simulink model "safir_a"  (R2012b)
(part 2 of 48)

      | port_label('input', 1, 'd');
      | port_label('output', 1, 'q');
      | disp(['Z^-', num2str(latency)]);
  pipeline77 : Subsystem  AncestorBlock=casper_library_delays/pipeline  mask(pipeline){latency=2}
      mask help:
      | An explicitly laid-out delay line to avoid mapping to SRL16s
      | for use in pipelining to help achieve timing closure.
      mask init:
      | pipeline_init(gcb,'latency',latency);
      settings: AttributesFormatString=Latency = %<latency>
      mask Display:
      | port_label('input', 1, 'd');
      | port_label('output', 1, 'q');
      | disp(['Z^-', num2str(latency)]);
  pipeline8 : Subsystem  AncestorBlock=casper_library_delays/pipeline  mask(pipeline){latency=2}
      mask help:
      | An explicitly laid-out delay line to avoid mapping to SRL16s
      | for use in pipelining to help achieve timing closure.
      mask init:
      | pipeline_init(gcb,'latency',latency);
      settings: AttributesFormatString=Latency = %<latency>
      mask Display:
      | port_label('input', 1, 'd');
      | port_label('output', 1, 'q');
      | disp(['Z^-', num2str(latency)]);
  pipeline9 : Subsystem  AncestorBlock=casper_library_delays/pipeline  mask(pipeline){latency=2}
      mask help:
      | An explicitly laid-out delay line to avoid mapping to SRL16s
      | for use in pipelining to help achieve timing closure.
      mask init:
      | pipeline_init(gcb,'latency',latency);
      settings: AttributesFormatString=Latency = %<latency>
      mask Display:
      | port_label('input', 1, 'd');
      | port_label('output', 1, 'q');
      | disp(['Z^-', num2str(latency)]);
  receptor_id : Subsystem  Tag=xps:sw_reg  AncestorBlock=xps_library/software register  mask(swreg){mode=fields of arbitrary size, io_dir=From Processor, io_delay=1, sample_period=1, names=[receptor_id pol0_id pol1_id], bitwidths=[14 2 2], arith_types=[0 0 0], bin_pts=[0 0 0], show_format=on}
      mask prompts: io_dir "I/O direction"; io_delay "I/O delay"; sample_period "Sample period"; names "Names [msb ... lsb]:"; bitwidths "Bitwidths [msb ... lsb]:"; arith_types "Types (ufix=0, fix=1, bool=2) [msb ... lsb]:"; bin_pts "Binary pts [msb ... lsb]:"; show_format "Print format string?"
      mask init:
      | swreg_init(gcb)
      settings: AttributesFormatString=3 inputs:uf14.0,uf2.0,uf2.0,
      mask TypeOptions mode: one value | fields of equal size | fields of arbitrary size
      mask Callback mode: swreg_cb(gcb);
      mask TypeOptions io_dir: To Processor | From Processor
      mask Callback io_dir:
      | mask_enables = get_param(gcb, 'MaskEnables');
      | mask_names = get_param(gcb, 'MaskNames');
      | if strcmp(get_param(gcb, 'io_dir'), 'To Processor'),
      |     mask_enables{ismember(mask_names, 'sample_period')} = 'off';
      | else
      |     mask_enables{ismember(mask_names, 'sample_period')} = 'on';
      | end
      | set_param(gcb, 'MaskEnables', mask_enables);
      mask Callback bitwidths:
      | blk = gcb;
      | mode = get_param(blk, 'mode');
      | current_widths = eval(get_param(blk, 'bitwidths'));
      | if (strcmp(mode, 'one value') || strcmp(mode, 'fields of equal size')) && (length(current_widths) > 1),
      |     error('Only one width may be specified for this mode.');
      | elseif strcmp(mode, 'fields of arbitrary size')
      |     current_names = textscan(strtrim(strrep(strrep(get_param(blk, 'names'), ']', ''), '[', '')), '%s');
      |     current_names = current_names{1};
      |     numios = length(current_names);
      |     if length(current_widths) ~= numios,
      |         error('%d field names specified, but %d widths?', numios, length(current_widths));
      |     end
      | end
      | total_width = 0;
      | for ctr = 1 : length(current_widths),
      |     total_width = total_width + current_widths(ctr);
      | end
      | if total_width > 32,
      |     error('Total width must be 32 or less, set to %d.', total_width);
      | end
      mask Callback arith_types:
      | blk = gcb;
      | mode = get_param(blk, 'mode');
      | current_types = eval(get_param(blk, 'arith_types'));
      | numios = length(current_types);
      | if (strcmp(mode, 'one value') || strcmp(mode, 'fields of equal size')) && (length(current_types) > 1),
      |     error('Only one type may be specified for this mode.');
      | elseif strcmp(mode, 'fields of arbitrary size')
      |     current_names = textscan(strtrim(strrep(strrep(get_param(blk, 'names'), ']', ''), '[', '')), '%s');
      |     current_names = current_names{1};
      |     numios = length(current_names);
      |     if length(current_types) ~= numios,
      |         error('%d field names specified, but %d types?', numios, length(current_types));
      |     end
      | end
      | problem = 0;
      | for ctr = 1 : numios,
      |     t = current_types(ctr);
      |     if (t < 0) || (t > 2),
      |         problem = t;
      |         ctr = numios + 1;
      |     end
      | end
      | if problem ~= 0,
      |     error('Type cannot be %i, must be 0, 1 or 2.', problem);
      | end
      mask Callback bin_pts:
      | blk = gcb;
      | mode = get_param(blk, 'mode');
      | current_bins = eval(get_param(blk, 'bin_pts'));
      | if (strcmp(mode, 'one value') || strcmp(mode, 'fields of equal size')) && (length(current_bins) > 1),
      |     error('Only one binary pt may be specified for this mode.');
      | elseif strcmp(mode, 'fields of arbitrary size')
      |     current_names = textscan(strtrim(strrep(strrep(get_param(blk, 'names'), ']', ''), '[', '')), '%s');
      |     current_names = current_names{1};
      |     numios = length(current_names);
      |     if length(current_bins) ~= numios,
      |         error('%d field names specified, but %d binary pts?', numios, length(current_bins));
      |     end
      | end
  recverr_ctr : Subsystem  Tag=xps:sw_reg  AncestorBlock=xps_library/software register  mask(swreg){mode=fields of equal size, io_dir=To Processor, io_delay=0, sample_period=1, names=[p0 p1], bitwidths=16, arith_types=0, bin_pts=0, sim_port=off, show_format=on}
      mask prompts: io_dir "I/O direction"; io_delay "I/O delay"; sample_period "Sample period"; names "Names [msb ... lsb]:"; bitwidths "Bitwidth:"; arith_types "Type (ufix=0, fix=1, bool=2):"; bin_pts "Binary pt:"; sim_port "Provide sim input/output?"; show_format "Print format string?"
      mask init:
      | swreg_init(gcb)
      settings: AttributesFormatString=2 outputs:uf16.0,uf16.0,
      mask TypeOptions mode: one value | fields of equal size | fields of arbitrary size
      mask Callback mode: swreg_cb(gcb);
      mask TypeOptions io_dir: To Processor | From Processor
      mask Callback io_dir:
      | mask_enables = get_param(gcb, 'MaskEnables');
      | mask_names = get_param(gcb, 'MaskNames');
      | if strcmp(get_param(gcb, 'io_dir'), 'To Processor'),
      |     mask_enables{ismember(mask_names, 'sample_period')} = 'off';
      | else
      |     mask_enables{ismember(mask_names, 'sample_period')} = 'on';
      | end
      | set_param(gcb, 'MaskEnables', mask_enables);
      mask Callback bitwidths:
      | blk = gcb;
      | mode = get_param(blk, 'mode');
      | current_widths = eval(get_param(blk, 'bitwidths'));
      | if (strcmp(mode, 'one value') || strcmp(mode, 'fields of equal size')) && (length(current_widths) > 1),
      |     error('Only one width may be specified for this mode.');
      | elseif strcmp(mode, 'fields of arbitrary size')
      |     current_names = textscan(strtrim(strrep(strrep(get_param(blk, 'names'), ']', ''), '[', '')), '%s');
      |     current_names = current_names{1};
      |     numios = length(current_names);
      |     if length(current_widths) ~= numios,
      |         error('%d field names specified, but %d widths?', numios, length(current_widths));
      |     end
      | end
      | total_width = 0;
      | for ctr = 1 : length(current_widths),
      |     total_width = total_width + current_widths(ctr);
      | end
      | if total_width > 32,
      |     error('Total width must be 32 or less, set to %d.', total_width);
      | end
      mask Callback arith_types:
      | blk = gcb;
      | mode = get_param(blk, 'mode');
      | current_types = eval(get_param(blk, 'arith_types'));
      | numios = length(current_types);
      | if (strcmp(mode, 'one value') || strcmp(mode, 'fields of equal size')) && (length(current_types) > 1),
      |     error('Only one type may be specified for this mode.');
      | elseif strcmp(mode, 'fields of arbitrary size')
      |     current_names = textscan(strtrim(strrep(strrep(get_param(blk, 'names'), ']', ''), '[', '')), '%s');
      |     current_names = current_names{1};
      |     numios = length(current_names);
      |     if length(current_types) ~= numios,
      |         error('%d field names specified, but %d types?', numios, length(current_types));
      |     end
      | end
      | problem = 0;
      | for ctr = 1 : numios,
      |     t = current_types(ctr);
      |     if (t < 0) || (t > 2),
      |         problem = t;
      |         ctr = numios + 1;
      |     end
      | end
      | if problem ~= 0,
      |     error('Type cannot be %i, must be 0, 1 or 2.', problem);
      | end
      mask Callback bin_pts:
      | blk = gcb;
      | mode = get_param(blk, 'mode');
      | current_bins = eval(get_param(blk, 'bin_pts'));
      | if (strcmp(mode, 'one value') || strcmp(mode, 'fields of equal size')) && (length(current_bins) > 1),
      |     error('Only one binary pt may be specified for this mode.');
      | elseif strcmp(mode, 'fields of arbitrary size')
      |     current_names = textscan(strtrim(strrep(strrep(get_param(blk, 'names'), ']', ''), '[', '')), '%s');
      |     current_names = current_names{1};
      |     numios = length(current_names);
      |     if length(current_bins) ~= numios,
      |         error('%d field names specified, but %d binary pts?', numios, length(current_bins));
      |     end
      | end
  serial_to_8par : Subsystem
  serial_to_8par1 : Subsystem
  slice1 : xbsIndex_r4/Slice  nbits=2  boolean_output=off  mode=Two Bit Locations  bit1=0  base1=MSB of Input  bit0=3  base0=LSB of Input  dbl_ovrd=off  block_type=slice
  spead_pack0 : Subsystem  Tag=casper:spead_pack  AncestorBlock=casper_library_communications/spead_pack  mask(pkt_pack_mask){max_pkt_len_bits=10, header_ids=0x1600, 0x3101, 0x3102, header_ind_ids=0x3300, spead_msw=64, spead_lsw=48, spead_version=4, bytes_per_word=8}
      mask prompts: max_pkt_len_bits "Max pkt length, 2^? 64-bit words"; header_ids "SPEAD direct address IDs (decimal)"; header_ind_ids "SPEAD indirect address IDs (decimal)"; spead_msw "SPEAD Flavour (MSw)"; spead_lsw "SPEAD Flavour (LSw)"; spead_version "SPEAD version"; bytes_per_word "Word size, in bytes"
      mask help:
      | This block generates SPEAD-compliant packets from a datastream.
      |
      | Packets are created with a fixed header followed by a number of 64-bit items.
      |
      | Requires a 64-bit data stream.
      |
      | The data_ready signal is one cycle BEFORE valid data! Does not have to be with a valid signal either.
      mask init:
      | if floor(log2(bytes_per_word)) ~= log2(bytes_per_word)
      |     error('Bytes per word should be a power of two.');
      | end
      | 
      | spead_pack_init(gcb)
  spead_pack1 : Subsystem  Tag=casper:spead_pack  AncestorBlock=casper_library_communications/spead_pack  mask(pkt_pack_mask){max_pkt_len_bits=10, header_ids=0x1600, 0x3101, 0x3102, header_ind_ids=0x3300, spead_msw=64, spead_lsw=48, spead_version=4, bytes_per_word=8}
      mask prompts: max_pkt_len_bits "Max pkt length, 2^? 64-bit words"; header_ids "SPEAD direct address IDs (decimal)"; header_ind_ids "SPEAD indirect address IDs (decimal)"; spead_msw "SPEAD Flavour (MSw)"; spead_lsw "SPEAD Flavour (LSw)"; spead_version "SPEAD version"; bytes_per_word "Word size, in bytes"
      mask help:
      | This block generates SPEAD-compliant packets from a datastream.
      |
      | Packets are created with a fixed header followed by a number of 64-bit items.
      |
      | Requires a 64-bit data stream.
      |
      | The data_ready signal is one cycle BEFORE valid data! Does not have to be with a valid signal either.
      mask init:
      | if floor(log2(bytes_per_word)) ~= log2(bytes_per_word)
      |     error('Bytes per word should be a power of two.');
      | end
      | 
      | spead_pack_init(gcb)
  spead_pack2 : Subsystem  Tag=casper:spead_pack  AncestorBlock=casper_library_communications/spead_pack  mask(pkt_pack_mask){max_pkt_len_bits=10, header_ids=0x1600, 0x3101, 0x3102, header_ind_ids=0x3300, spead_msw=64, spead_lsw=48, spead_version=4, bytes_per_word=8}
      mask prompts: max_pkt_len_bits "Max pkt length, 2^? 64-bit words"; header_ids "SPEAD direct address IDs (decimal)"; header_ind_ids "SPEAD indirect address IDs (decimal)"; spead_msw "SPEAD Flavour (MSw)"; spead_lsw "SPEAD Flavour (LSw)"; spead_version "SPEAD version"; bytes_per_word "Word size, in bytes"
      mask help:
      | This block generates SPEAD-compliant packets from a datastream.
      |
      | Packets are created with a fixed header followed by a number of 64-bit items.
      |
      | Requires a 64-bit data stream.
      |
      | The data_ready signal is one cycle BEFORE valid data! Does not have to be with a valid signal either.
      mask init:
      | if floor(log2(bytes_per_word)) ~= log2(bytes_per_word)
      |     error('Bytes per word should be a power of two.');
      | end
      | 
      | spead_pack_init(gcb)
  spead_pack3 : Subsystem  Tag=casper:spead_pack  AncestorBlock=casper_library_communications/spead_pack  mask(pkt_pack_mask){max_pkt_len_bits=10, header_ids=0x1600, 0x3101, 0x3102, header_ind_ids=0x3300, spead_msw=64, spead_lsw=48, spead_version=4, bytes_per_word=8}
      mask prompts: max_pkt_len_bits "Max pkt length, 2^? 64-bit words"; header_ids "SPEAD direct address IDs (decimal)"; header_ind_ids "SPEAD indirect address IDs (decimal)"; spead_msw "SPEAD Flavour (MSw)"; spead_lsw "SPEAD Flavour (LSw)"; spead_version "SPEAD version"; bytes_per_word "Word size, in bytes"
      mask help:
      | This block generates SPEAD-compliant packets from a datastream.
      |
      | Packets are created with a fixed header followed by a number of 64-bit items.
      |
      | Requires a 64-bit data stream.
      |
      | The data_ready signal is one cycle BEFORE valid data! Does not have to be with a valid signal either.
      mask init:
      | if floor(log2(bytes_per_word)) ~= log2(bytes_per_word)
      |     error('Bytes per word should be a power of two.');
      | end
      | 
      | spead_pack_init(gcb)
  sync_gen : Subsystem  mask{zerolsbs=((15 + 1) + 8) - 12}
      mask prompts: zerolsbs "No. LSBs to be zero:"
  sync_timestamp_lsw : Subsystem  Tag=xps:sw_reg  AncestorBlock=xps_library/software register  mask(swreg){mode=fields of arbitrary size, io_dir=To Processor, io_delay=0, sample_period=1, names=[time_lsw pkt_size tstep_err_ctr sync80_ctr valid80_ctr], bitwidths=[4 10 6 6 6], arith_types=[0 0 0 0 0], bin_pts=[0 0 0 0 0], sim_port=off, show_format=on}
      mask prompts: io_dir "I/O direction"; io_delay "I/O delay"; sample_period "Sample period"; names "Names [msb ... lsb]:"; bitwidths "Bitwidths [msb ... lsb]:"; arith_types "Types (ufix=0, fix=1, bool=2) [msb ... lsb]:"; bin_pts "Binary pts [msb ... lsb]:"; sim_port "Provide sim input/output?"; show_format "Print format string?"
      mask init:
      | swreg_init(gcb)
      settings: AttributesFormatString=5 outputs:uf4.0,uf10.0,uf6.0,uf6.0,uf6.0,
      mask TypeOptions mode: one value | fields of equal size | fields of arbitrary size
      mask Callback mode: swreg_cb(gcb);
      mask TypeOptions io_dir: To Processor | From Processor
      mask Callback io_dir:
      | mask_enables = get_param(gcb, 'MaskEnables');
      | mask_names = get_param(gcb, 'MaskNames');
      | if strcmp(get_param(gcb, 'io_dir'), 'To Processor'),
      |     mask_enables{ismember(mask_names, 'sample_period')} = 'off';
      | else
      |     mask_enables{ismember(mask_names, 'sample_period')} = 'on';
      | end
      | set_param(gcb, 'MaskEnables', mask_enables);
      mask Callback bitwidths:
      | blk = gcb;
      | mode = get_param(blk, 'mode');
      | current_widths = eval(get_param(blk, 'bitwidths'));
      | if (strcmp(mode, 'one value') || strcmp(mode, 'fields of equal size')) && (length(current_widths) > 1),
      |     error('Only one width may be specified for this mode.');
      | elseif strcmp(mode, 'fields of arbitrary size')
      |     current_names = textscan(strtrim(strrep(strrep(get_param(blk, 'names'), ']', ''), '[', '')), '%s');
      |     current_names = current_names{1};
      |     numios = length(current_names);
      |     if length(current_widths) ~= numios,
      |         error('%d field names specified, but %d widths?', numios, length(current_widths));
      |     end
      | end
      | total_width = 0;
      | for ctr = 1 : length(current_widths),
      |     total_width = total_width + current_widths(ctr);
      | end
      | if total_width > 32,
      |     error('Total width must be 32 or less, set to %d.', total_width);
      | end
      mask Callback arith_types:
      | blk = gcb;
      | mode = get_param(blk, 'mode');
      | current_types = eval(get_param(blk, 'arith_types'));
      | numios = length(current_types);
      | if (strcmp(mode, 'one value') || strcmp(mode, 'fields of equal size')) && (length(current_types) > 1),
      |     error('Only one type may be specified for this mode.');
      | elseif strcmp(mode, 'fields of arbitrary size')
      |     current_names = textscan(strtrim(strrep(strrep(get_param(blk, 'names'), ']', ''), '[', '')), '%s');
      |     current_names = current_names{1};
      |     numios = length(current_names);
      |     if length(current_types) ~= numios,
      |         error('%d field names specified, but %d types?', numios, length(current_types));
      |     end
      | end
      | problem = 0;
      | for ctr = 1 : numios,
      |     t = current_types(ctr);
      |     if (t < 0) || (t > 2),
      |         problem = t;
      |         ctr = numios + 1;
      |     end
      | end
      | if problem ~= 0,
      |     error('Type cannot be %i, must be 0, 1 or 2.', problem);
      | end
      mask Callback bin_pts:
      | blk = gcb;
      | mode = get_param(blk, 'mode');
      | current_bins = eval(get_param(blk, 'bin_pts'));
      | if (strcmp(mode, 'one value') || strcmp(mode, 'fields of equal size')) && (length(current_bins) > 1),
      |     error('Only one binary pt may be specified for this mode.');
      | elseif strcmp(mode, 'fields of arbitrary size')
      |     current_names = textscan(strtrim(strrep(strrep(get_param(blk, 'names'), ']', ''), '[', '')), '%s');
      |     current_names = current_names{1};
      |     numios = length(current_names);
      |     if length(current_bins) ~= numios,
      |         error('%d field names specified, but %d binary pts?', numios, length(current_bins));
      |     end
      | end
  sync_timestamp_msw : Subsystem  Tag=xps:sw_reg  AncestorBlock=xps_library/software register  mask(swreg){mode=one value, io_dir=To Processor, io_delay=0, sample_period=1, names=reg, bitwidths=32, arith_types=0, bin_pts=0, sim_port=off, show_format=on}
      mask prompts: io_dir "I/O direction"; io_delay "I/O delay"; sample_period "Sample period"; names "Name:"; bitwidths "Bitwidth:"; arith_types "Type (ufix=0, fix=1, bool=2):"; bin_pts "Binary pt:"; sim_port "Provide sim input/output?"; show_format "Print format string?"
      mask init:
      | swreg_init(gcb)
      settings: AttributesFormatString=1output:uf32.0,
      mask TypeOptions mode: one value | fields of equal size | fields of arbitrary size
      mask Callback mode: swreg_cb(gcb);
      mask TypeOptions io_dir: To Processor | From Processor
      mask Callback io_dir:
      | mask_enables = get_param(gcb, 'MaskEnables');
      | mask_names = get_param(gcb, 'MaskNames');
      | if strcmp(get_param(gcb, 'io_dir'), 'To Processor'),
      |     mask_enables{ismember(mask_names, 'sample_period')} = 'off';
      | else
      |     mask_enables{ismember(mask_names, 'sample_period')} = 'on';
      | end
      | set_param(gcb, 'MaskEnables', mask_enables);
      mask Callback bitwidths:
      | blk = gcb;
      | mode = get_param(blk, 'mode');
      | current_widths = eval(get_param(blk, 'bitwidths'));
      | if (strcmp(mode, 'one value') || strcmp(mode, 'fields of equal size')) && (length(current_widths) > 1),
      |     error('Only one width may be specified for this mode.');
      | elseif strcmp(mode, 'fields of arbitrary size')
      |     current_names = textscan(strtrim(strrep(strrep(get_param(blk, 'names'), ']', ''), '[', '')), '%s');
      |     current_names = current_names{1};
      |     numios = length(current_names);
      |     if length(current_widths) ~= numios,
      |         error('%d field names specified, but %d widths?', numios, length(current_widths));
      |     end
      | end
      | total_width = 0;
      | for ctr = 1 : length(current_widths),
      |     total_width = total_width + current_widths(ctr);
      | end
      | if total_width > 32,
      |     error('Total width must be 32 or less, set to %d.', total_width);
      | end
      mask Callback arith_types:
      | blk = gcb;
      | mode = get_param(blk, 'mode');
      | current_types = eval(get_param(blk, 'arith_types'));
      | numios = length(current_types);
      | if (strcmp(mode, 'one value') || strcmp(mode, 'fields of equal size')) && (length(current_types) > 1),
      |     error('Only one type may be specified for this mode.');
      | elseif strcmp(mode, 'fields of arbitrary size')
      |     current_names = textscan(strtrim(strrep(strrep(get_param(blk, 'names'), ']', ''), '[', '')), '%s');
      |     current_names = current_names{1};
      |     numios = length(current_names);
      |     if length(current_types) ~= numios,
      |         error('%d field names specified, but %d types?', numios, length(current_types));
      |     end
      | end
      | problem = 0;
      | for ctr = 1 : numios,
      |     t = current_types(ctr);
      |     if (t < 0) || (t > 2),
      |         problem = t;
      |         ctr = numios + 1;
      |     end
      | end
      | if problem ~= 0,
      |     error('Type cannot be %i, must be 0, 1 or 2.', problem);
      | end
      mask Callback bin_pts:
      | blk = gcb;
      | mode = get_param(blk, 'mode');
      | current_bins = eval(get_param(blk, 'bin_pts'));
      | if (strcmp(mode, 'one value') || strcmp(mode, 'fields of equal size')) && (length(current_bins) > 1),
      |     error('Only one binary pt may be specified for this mode.');
      | elseif strcmp(mode, 'fields of arbitrary size')
      |     current_names = textscan(strtrim(strrep(strrep(get_param(blk, 'names'), ']', ''), '[', '')), '%s');
      |     current_names = current_names{1};
      |     numios = length(current_names);
      |     if length(current_bins) ~= numios,
      |         error('%d field names specified, but %d binary pts?', numios, length(current_bins));
      |     end
      | end
  timestep_ages : Subsystem  Tag=xps:sw_reg  AncestorBlock=xps_library/software register  mask(swreg){mode=fields of equal size, io_dir=To Processor, io_delay=0, sample_period=1, names=[future past], bitwidths=16, arith_types=0, bin_pts=0, sim_port=off, show_format=on}
      mask prompts: io_dir "I/O direction"; io_delay "I/O delay"; sample_period "Sample period"; names "Names [msb ... lsb]:"; bitwidths "Bitwidth:"; arith_types "Type (ufix=0, fix=1, bool=2):"; bin_pts "Binary pt:"; sim_port "Provide sim input/output?"; show_format "Print format string?"
      mask init:
      | swreg_init(gcb)
      settings: AttributesFormatString=2 outputs:uf16.0,uf16.0,
      mask TypeOptions mode: one value | fields of equal size | fields of arbitrary size
      mask Callback mode: swreg_cb(gcb);
      mask TypeOptions io_dir: To Processor | From Processor
      mask Callback io_dir:
      | mask_enables = get_param(gcb, 'MaskEnables');
      | mask_names = get_param(gcb, 'MaskNames');
      | if strcmp(get_param(gcb, 'io_dir'), 'To Processor'),
      |     mask_enables{ismember(mask_names, 'sample_period')} = 'off';
      | else
      |     mask_enables{ismember(mask_names, 'sample_period')} = 'on';
      | end
      | set_param(gcb, 'MaskEnables', mask_enables);
      mask Callback bitwidths:
      | blk = gcb;
      | mode = get_param(blk, 'mode');
      | current_widths = eval(get_param(blk, 'bitwidths'));
      | if (strcmp(mode, 'one value') || strcmp(mode, 'fields of equal size')) && (length(current_widths) > 1),
      |     error('Only one width may be specified for this mode.');
      | elseif strcmp(mode, 'fields of arbitrary size')
      |     current_names = textscan(strtrim(strrep(strrep(get_param(blk, 'names'), ']', ''), '[', '')), '%s');
      |     current_names = current_names{1};
      |     numios = length(current_names);
      |     if length(current_widths) ~= numios,
      |         error('%d field names specified, but %d widths?', numios, length(current_widths));
      |     end
      | end
      | total_width = 0;
      | for ctr = 1 : length(current_widths),
      |     total_width = total_width + current_widths(ctr);
      | end
      | if total_width > 32,
      |     error('Total width must be 32 or less, set to %d.', total_width);
      | end
      mask Callback arith_types:
      | blk = gcb;
      | mode = get_param(blk, 'mode');
      | current_types = eval(get_param(blk, 'arith_types'));
      | numios = length(current_types);
      | if (strcmp(mode, 'one value') || strcmp(mode, 'fields of equal size')) && (length(current_types) > 1),
      |     error('Only one type may be specified for this mode.');
      | elseif strcmp(mode, 'fields of arbitrary size')
      |     current_names = textscan(strtrim(strrep(strrep(get_param(blk, 'names'), ']', ''), '[', '')), '%s');
      |     current_names = current_names{1};
      |     numios = length(current_names);
      |     if length(current_types) ~= numios,
      |         error('%d field names specified, but %d types?', numios, length(current_types));
      |     end
      | end
      | problem = 0;
      | for ctr = 1 : numios,
      |     t = current_types(ctr);
      |     if (t < 0) || (t > 2),
      |         problem = t;
      |         ctr = numios + 1;
      |     end
      | end
      | if problem ~= 0,
      |     error('Type cannot be %i, must be 0, 1 or 2.', problem);
      | end
      mask Callback bin_pts:
      | blk = gcb;
      | mode = get_param(blk, 'mode');
      | current_bins = eval(get_param(blk, 'bin_pts'));
      | if (strcmp(mode, 'one value') || strcmp(mode, 'fields of equal size')) && (length(current_bins) > 1),
      |     error('Only one binary pt may be specified for this mode.');
      | elseif strcmp(mode, 'fields of arbitrary size')
      |     current_names = textscan(strtrim(strrep(strrep(get_param(blk, 'names'), ']', ''), '[', '')), '%s');
      |     current_names = current_names{1};
      |     numios = length(current_names);
      |     if length(current_bins) ~= numios,
      |         error('%d field names specified, but %d binary pts?', numios, length(current_bins));
      |     end
      | end
  tmiss_ctr : Subsystem  Tag=xps:sw_reg  AncestorBlock=xps_library/software register  mask(swreg){mode=fields of equal size, io_dir=To Processor, io_delay=0, sample_period=1, names=[p0 p1], bitwidths=16, arith_types=0, bin_pts=0, sim_port=off, show_format=on}
      mask prompts: io_dir "I/O direction"; io_delay "I/O delay"; sample_period "Sample period"; names "Names [msb ... lsb]:"; bitwidths "Bitwidth:"; arith_types "Type (ufix=0, fix=1, bool=2):"; bin_pts "Binary pt:"; sim_port "Provide sim input/output?"; show_format "Print format string?"
      mask init:
      | swreg_init(gcb)
      settings: AttributesFormatString=2 outputs:uf16.0,uf16.0,
      mask TypeOptions mode: one value | fields of equal size | fields of arbitrary size
      mask Callback mode: swreg_cb(gcb);
      mask TypeOptions io_dir: To Processor | From Processor
      mask Callback io_dir:
      | mask_enables = get_param(gcb, 'MaskEnables');
      | mask_names = get_param(gcb, 'MaskNames');
      | if strcmp(get_param(gcb, 'io_dir'), 'To Processor'),
      |     mask_enables{ismember(mask_names, 'sample_period')} = 'off';
      | else
      |     mask_enables{ismember(mask_names, 'sample_period')} = 'on';
      | end
      | set_param(gcb, 'MaskEnables', mask_enables);
      mask Callback bitwidths:
      | blk = gcb;
      | mode = get_param(blk, 'mode');
      | current_widths = eval(get_param(blk, 'bitwidths'));
      | if (strcmp(mode, 'one value') || strcmp(mode, 'fields of equal size')) && (length(current_widths) > 1),
      |     error('Only one width may be specified for this mode.');
      | elseif strcmp(mode, 'fields of arbitrary size')
      |     current_names = textscan(strtrim(strrep(strrep(get_param(blk, 'names'), ']', ''), '[', '')), '%s');
      |     current_names = current_names{1};
      |     numios = length(current_names);
      |     if length(current_widths) ~= numios,
      |         error('%d field names specified, but %d widths?', numios, length(current_widths));
      |     end
      | end
      | total_width = 0;
      | for ctr = 1 : length(current_widths),
      |     total_width = total_width + current_widths(ctr);
      | end
      | if total_width > 32,
      |     error('Total width must be 32 or less, set to %d.', total_width);
      | end
      mask Callback arith_types:
      | blk = gcb;
      | mode = get_param(blk, 'mode');
      | current_types = eval(get_param(blk, 'arith_types'));
      | numios = length(current_types);
      | if (strcmp(mode, 'one value') || strcmp(mode, 'fields of equal size')) && (length(current_types) > 1),
      |     error('Only one type may be specified for this mode.');
      | elseif strcmp(mode, 'fields of arbitrary size')
      |     current_names = textscan(strtrim(strrep(strrep(get_param(blk, 'names'), ']', ''), '[', '')), '%s');
      |     current_names = current_names{1};
      |     numios = length(current_names);
      |     if length(current_types) ~= numios,
      |         error('%d field names specified, but %d types?', numios, length(current_types));
      |     end
      | end
      | problem = 0;
      | for ctr = 1 : numios,
      |     t = current_types(ctr);
      |     if (t < 0) || (t > 2),
      |         problem = t;
      |         ctr = numios + 1;
      |     end
      | end
      | if problem ~= 0,
      |     error('Type cannot be %i, must be 0, 1 or 2.', problem);
      | end
      mask Callback bin_pts:
      | blk = gcb;
      | mode = get_param(blk, 'mode');
      | current_bins = eval(get_param(blk, 'bin_pts'));
      | if (strcmp(mode, 'one value') || strcmp(mode, 'fields of equal size')) && (length(current_bins) > 1),
      |     error('Only one binary pt may be specified for this mode.');
      | elseif strcmp(mode, 'fields of arbitrary size')
      |     current_names = textscan(strtrim(strrep(strrep(get_param(blk, 'names'), ']', ''), '[', '')), '%s');
      |     current_names = current_names{1};
      |     numios = length(current_names);
      |     if length(current_bins) ~= numios,
      |         error('%d field names specified, but %d binary pts?', numios, length(current_bins));
      |     end
      | end
  tmiss_p0 : Subsystem  Tag=xps:sw_reg  AncestorBlock=xps_library/software register  mask(swreg){mode=one value, io_dir=To Processor, io_delay=0, sample_period=1, names=reg, bitwidths=32, arith_types=0, bin_pts=0, sim_port=off, show_format=on}
      mask prompts: io_dir "I/O direction"; io_delay "I/O delay"; sample_period "Sample period"; names "Name:"; bitwidths "Bitwidth:"; arith_types "Type (ufix=0, fix=1, bool=2):"; bin_pts "Binary pt:"; sim_port "Provide sim input/output?"; show_format "Print format string?"
      mask init:
      | swreg_init(gcb)
      settings: AttributesFormatString=1output:uf32.0,
      mask TypeOptions mode: one value | fields of equal size | fields of arbitrary size
      mask Callback mode: swreg_cb(gcb);
      mask TypeOptions io_dir: To Processor | From Processor
      mask Callback io_dir:
      | mask_enables = get_param(gcb, 'MaskEnables');
      | mask_names = get_param(gcb, 'MaskNames');
      | if strcmp(get_param(gcb, 'io_dir'), 'To Processor'),
      |     mask_enables{ismember(mask_names, 'sample_period')} = 'off';
      | else
      |     mask_enables{ismember(mask_names, 'sample_period')} = 'on';
      | end
      | set_param(gcb, 'MaskEnables', mask_enables);
      mask Callback bitwidths:
      | blk = gcb;
      | mode = get_param(blk, 'mode');
      | current_widths = eval(get_param(blk, 'bitwidths'));
      | if (strcmp(mode, 'one value') || strcmp(mode, 'fields of equal size')) && (length(current_widths) > 1),
      |     error('Only one width may be specified for this mode.');
      | elseif strcmp(mode, 'fields of arbitrary size')
      |     current_names = textscan(strtrim(strrep(strrep(get_param(blk, 'names'), ']', ''), '[', '')), '%s');
      |     current_names = current_names{1};
      |     numios = length(current_names);
      |     if length(current_widths) ~= numios,
      |         error('%d field names specified, but %d widths?', numios, length(current_widths));
      |     end
      | end
      | total_width = 0;
      | for ctr = 1 : length(current_widths),
      |     total_width = total_width + current_widths(ctr);
      | end
      | if total_width > 32,
      |     error('Total width must be 32 or less, set to %d.', total_width);
      | end
      mask Callback arith_types:
      | blk = gcb;
      | mode = get_param(blk, 'mode');
      | current_types = eval(get_param(blk, 'arith_types'));
      | numios = length(current_types);
      | if (strcmp(mode, 'one value') || strcmp(mode, 'fields of equal size')) && (length(current_types) > 1),
      |     error('Only one type may be specified for this mode.');
      | elseif strcmp(mode, 'fields of arbitrary size')
      |     current_names = textscan(strtrim(strrep(strrep(get_param(blk, 'names'), ']', ''), '[', '')), '%s');
      |     current_names = current_names{1};
      |     numios = length(current_names);
      |     if length(current_types) ~= numios,
      |         error('%d field names specified, but %d types?', numios, length(current_types));
      |     end
      | end
      | problem = 0;
      | for ctr = 1 : numios,
      |     t = current_types(ctr);
      |     if (t < 0) || (t > 2),
      |         problem = t;
      |         ctr = numios + 1;
      |     end
      | end
      | if problem ~= 0,
      |     error('Type cannot be %i, must be 0, 1 or 2.', problem);
      | end
      mask Callback bin_pts:
      | blk = gcb;
      | mode = get_param(blk, 'mode');
      | current_bins = eval(get_param(blk, 'bin_pts'));
      | if (strcmp(mode, 'one value') || strcmp(mode, 'fields of equal size')) && (length(current_bins) > 1),
      |     error('Only one binary pt may be specified for this mode.');
      | elseif strcmp(mode, 'fields of arbitrary size')
      |     current_names = textscan(strtrim(strrep(strrep(get_param(blk, 'names'), ']', ''), '[', '')), '%s');
      |     current_names = current_names{1};
      |     numios = length(current_names);
      |     if length(current_bins) ~= numios,
      |         error('%d field names specified, but %d binary pts?', numios, length(current_bins));
      |     end
      | end
  tmiss_p1 : Subsystem  Tag=xps:sw_reg  AncestorBlock=xps_library/software register  mask(swreg){mode=one value, io_dir=To Processor, io_delay=0, sample_period=1, names=reg, bitwidths=32, arith_types=0, bin_pts=0, sim_port=off, show_format=on}
      mask prompts: io_dir "I/O direction"; io_delay "I/O delay"; sample_period "Sample period"; names "Name:"; bitwidths "Bitwidth:"; arith_types "Type (ufix=0, fix=1, bool=2):"; bin_pts "Binary pt:"; sim_port "Provide sim input/output?"; show_format "Print format string?"
      mask init:
      | swreg_init(gcb)
      settings: AttributesFormatString=1output:uf32.0,
      mask TypeOptions mode: one value | fields of equal size | fields of arbitrary size
      mask Callback mode: swreg_cb(gcb);
      mask TypeOptions io_dir: To Processor | From Processor
      mask Callback io_dir:
      | mask_enables = get_param(gcb, 'MaskEnables');
      | mask_names = get_param(gcb, 'MaskNames');
      | if strcmp(get_param(gcb, 'io_dir'), 'To Processor'),
      |     mask_enables{ismember(mask_names, 'sample_period')} = 'off';
      | else
      |     mask_enables{ismember(mask_names, 'sample_period')} = 'on';
      | end
      | set_param(gcb, 'MaskEnables', mask_enables);
      mask Callback bitwidths:
      | blk = gcb;
      | mode = get_param(blk, 'mode');
      | current_widths = eval(get_param(blk, 'bitwidths'));
      | if (strcmp(mode, 'one value') || strcmp(mode, 'fields of equal size')) && (length(current_widths) > 1),
      |     error('Only one width may be specified for this mode.');
      | elseif strcmp(mode, 'fields of arbitrary size')
      |     current_names = textscan(strtrim(strrep(strrep(get_param(blk, 'names'), ']', ''), '[', '')), '%s');
      |     current_names = current_names{1};
      |     numios = length(current_names);
      |     if length(current_widths) ~= numios,
      |         error('%d field names specified, but %d widths?', numios, length(current_widths));
      |     end
      | end
      | total_width = 0;
      | for ctr = 1 : length(current_widths),
      |     total_width = total_width + current_widths(ctr);
      | end
      | if total_width > 32,
      |     error('Total width must be 32 or less, set to %d.', total_width);
      | end
      mask Callback arith_types:
      | blk = gcb;
      | mode = get_param(blk, 'mode');
      | current_types = eval(get_param(blk, 'arith_types'));
      | numios = length(current_types);
      | if (strcmp(mode, 'one value') || strcmp(mode, 'fields of equal size')) && (length(current_types) > 1),
      |     error('Only one type may be specified for this mode.');
      | elseif strcmp(mode, 'fields of arbitrary size')
      |     current_names = textscan(strtrim(strrep(strrep(get_param(blk, 'names'), ']', ''), '[', '')), '%s');
      |     current_names = current_names{1};
      |     numios = length(current_names);
      |     if length(current_types) ~= numios,
      |         error('%d field names specified, but %d types?', numios, length(current_types));
      |     end
      | end
      | problem = 0;
      | for ctr = 1 : numios,
      |     t = current_types(ctr);
      |     if (t < 0) || (t > 2),
      |         problem = t;
      |         ctr = numios + 1;
      |     end
      | end
      | if problem ~= 0,
      |     error('Type cannot be %i, must be 0, 1 or 2.', problem);
      | end
      mask Callback bin_pts:
      | blk = gcb;
      | mode = get_param(blk, 'mode');
      | current_bins = eval(get_param(blk, 'bin_pts'));
      | if (strcmp(mode, 'one value') || strcmp(mode, 'fields of equal size')) && (length(current_bins) > 1),
      |     error('Only one binary pt may be specified for this mode.');
      | elseif strcmp(mode, 'fields of arbitrary size')
      |     current_names = textscan(strtrim(strrep(strrep(get_param(blk, 'names'), ']', ''), '[', '')), '%s');
      |     current_names = current_names{1};
      |     numios = length(current_names);
      |     if length(current_bins) ~= numios,
      |         error('%d field names specified, but %d binary pts?', numios, length(current_bins));
      |     end
      | end
  tvgsel : Subsystem  Tag=xps:sw_reg  AncestorBlock=xps_library/software register  mask(swreg){mode=fields of arbitrary size, io_dir=From Processor, io_delay=1, sample_period=1, names=[tvgsel field2], bitwidths=2, arith_types=0, bin_pts=0, show_format=on}
      mask prompts: io_dir "I/O direction"; io_delay "I/O delay"; sample_period "Sample period"; names "Names [msb ... lsb]:"; bitwidths "Bitwidths [msb ... lsb]:"; arith_types "Types (ufix=0, fix=1, bool=2) [msb ... lsb]:"; bin_pts "Binary pts [msb ... lsb]:"; show_format "Print format string?"
      mask init:
      | swreg_init(gcb)
      settings: AttributesFormatString=2 inputs:uf2.0,uf2.0,
      mask TypeOptions mode: one value | fields of equal size | fields of arbitrary size
      mask Callback mode: swreg_cb(gcb);
      mask TypeOptions io_dir: To Processor | From Processor
      mask Callback io_dir:
      | mask_enables = get_param(gcb, 'MaskEnables');
      | mask_names = get_param(gcb, 'MaskNames');
      | if strcmp(get_param(gcb, 'io_dir'), 'To Processor'),
      |     mask_enables{ismember(mask_names, 'sample_period')} = 'off';
      | else
      |     mask_enables{ismember(mask_names, 'sample_period')} = 'on';
      | end
      | set_param(gcb, 'MaskEnables', mask_enables);
      mask Callback bitwidths:
      | blk = gcb;
      | mode = get_param(blk, 'mode');
      | current_widths = eval(get_param(blk, 'bitwidths'));
      | if (strcmp(mode, 'one value') || strcmp(mode, 'fields of equal size')) && (length(current_widths) > 1),
      |     error('Only one width may be specified for this mode.');
      | elseif strcmp(mode, 'fields of arbitrary size')
      |     current_names = textscan(strtrim(strrep(strrep(get_param(blk, 'names'), ']', ''), '[', '')), '%s');
      |     current_names = current_names{1};
      |     numios = length(current_names);
      |     if length(current_widths) ~= numios,
      |         error('%d field names specified, but %d widths?', numios, length(current_widths));
      |     end
      | end
      | total_width = 0;
      | for ctr = 1 : length(current_widths),
      |     total_width = total_width + current_widths(ctr);
      | end
      | if total_width > 32,
      |     error('Total width must be 32 or less, set to %d.', total_width);
      | end
      mask Callback arith_types:
      | blk = gcb;
      | mode = get_param(blk, 'mode');
      | current_types = eval(get_param(blk, 'arith_types'));
      | numios = length(current_types);
      | if (strcmp(mode, 'one value') || strcmp(mode, 'fields of equal size')) && (length(current_types) > 1),
      |     error('Only one type may be specified for this mode.');
      | elseif strcmp(mode, 'fields of arbitrary size')
      |     current_names = textscan(strtrim(strrep(strrep(get_param(blk, 'names'), ']', ''), '[', '')), '%s');
      |     current_names = current_names{1};
      |     numios = length(current_names);
      |     if length(current_types) ~= numios,
      |         error('%d field names specified, but %d types?', numios, length(current_types));
      |     end
      | end
      | problem = 0;
      | for ctr = 1 : numios,
      |     t = current_types(ctr);
      |     if (t < 0) || (t > 2),
      |         problem = t;
      |         ctr = numios + 1;
      |     end
      | end
      | if problem ~= 0,
      |     error('Type cannot be %i, must be 0, 1 or 2.', problem);
      | end
      mask Callback bin_pts:
      | blk = gcb;
      | mode = get_param(blk, 'mode');
      | current_bins = eval(get_param(blk, 'bin_pts'));
      | if (strcmp(mode, 'one value') || strcmp(mode, 'fields of equal size')) && (length(current_bins) > 1),
      |     error('Only one binary pt may be specified for this mode.');
      | elseif strcmp(mode, 'fields of arbitrary size')
      |     current_names = textscan(strtrim(strrep(strrep(get_param(blk, 'names'), ']', ''), '[', '')), '%s');
      |     current_names = current_names{1};
      |     numios = length(current_names);
      |     if length(current_bins) ~= numios,
      |         error('%d field names specified, but %d binary pts?', numios, length(current_bins));
      |     end
      | end
  unpack_and_reorder : Subsystem  mask{n_bits_packet_size=9, n_bits_timestep=9+3, n_bits_fifo_depth=3, n_bits_buffer_depth=3, bram_latency=1}
      mask prompts: n_bits_packet_size "Packet size (2^? 80-bit words after unpacking)"; n_bits_timestep "Packet timestep (2^?)"; n_bits_fifo_depth "FIFO depth (2^? packets)"; n_bits_buffer_depth "Reorder buffer size (2^? packets)"; bram_latency "BRAM latency"
  up_debug : Subsystem  Tag=xps:sw_reg  AncestorBlock=xps_library/software register  mask(swreg){mode=one value, io_dir=From Processor, io_delay=0, sample_period=1, names=gbe_timestep, bitwidths=3, arith_types=0, bin_pts=0, sim_port=off, show_format=on}
      mask prompts: io_dir "I/O direction"; io_delay "I/O delay"; sample_period "Sample period"; names "Name:"; bitwidths "Bitwidth:"; arith_types "Type (ufix=0, fix=1, bool=2):"; bin_pts "Binary pt:"; sim_port "Provide sim input/output?"; show_format "Print format string?"
      mask init:
      | swreg_init(gcb)
      settings: AttributesFormatString=1input:uf3.0,
      mask TypeOptions mode: one value | fields of equal size | fields of arbitrary size
      mask Callback mode: swreg_cb(gcb);
      mask TypeOptions io_dir: To Processor | From Processor
      mask Callback io_dir:
      | mask_enables = get_param(gcb, 'MaskEnables');
      | mask_names = get_param(gcb, 'MaskNames');
      | if strcmp(get_param(gcb, 'io_dir'), 'To Processor'),
      |     mask_enables{ismember(mask_names, 'sample_period')} = 'off';
      | else
      |     mask_enables{ismember(mask_names, 'sample_period')} = 'on';
      | end
      | set_param(gcb, 'MaskEnables', mask_enables);
      mask Callback bitwidths:
      | blk = gcb;
      | mode = get_param(blk, 'mode');
      | current_widths = eval(get_param(blk, 'bitwidths'));
      | if (strcmp(mode, 'one value') || strcmp(mode, 'fields of equal size')) && (length(current_widths) > 1),
      |     error('Only one width may be specified for this mode.');
      | elseif strcmp(mode, 'fields of arbitrary size')
      |     current_names = textscan(strtrim(strrep(strrep(get_param(blk, 'names'), ']', ''), '[', '')), '%s');
      |     current_names = current_names{1};
      |     numios = length(current_names);
      |     if length(current_widths) ~= numios,
      |         error('%d field names specified, but %d widths?', numios, length(current_widths));
      |     end
      | end
      | total_width = 0;
      | for ctr = 1 : length(current_widths),
      |     total_width = total_width + current_widths(ctr);
      | end
      | if total_width > 32,
      |     error('Total width must be 32 or less, set to %d.', total_width);
      | end
      mask Callback arith_types:
      | blk = gcb;
      | mode = get_param(blk, 'mode');
      | current_types = eval(get_param(blk, 'arith_types'));
      | numios = length(current_types);
      | if (strcmp(mode, 'one value') || strcmp(mode, 'fields of equal size')) && (length(current_types) > 1),
      |     error('Only one type may be specified for this mode.');
      | elseif strcmp(mode, 'fields of arbitrary size')
      |     current_names = textscan(strtrim(strrep(strrep(get_param(blk, 'names'), ']', ''), '[', '')), '%s');
      |     current_names = current_names{1};
      |     numios = length(current_names);
      |     if length(current_types) ~= numios,
      |         error('%d field names specified, but %d types?', numios, length(current_types));
      |     end
      | end
      | problem = 0;
      | for ctr = 1 : numios,
      |     t = current_types(ctr);
      |     if (t < 0) || (t > 2),
      |         problem = t;
      |         ctr = numios + 1;
      |     end
      | end
      | if problem ~= 0,
      |     error('Type cannot be %i, must be 0, 1 or 2.', problem);
      | end
      mask Callback bin_pts:
      | blk = gcb;
      | mode = get_param(blk, 'mode');
      | current_bins = eval(get_param(blk, 'bin_pts'));
      | if (strcmp(mode, 'one value') || strcmp(mode, 'fields of equal size')) && (length(current_bins) > 1),
      |     error('Only one binary pt may be specified for this mode.');
      | elseif strcmp(mode, 'fields of arbitrary size')
      |     current_names = textscan(strtrim(strrep(strrep(get_param(blk, 'names'), ']', ''), '[', '')), '%s');
      |     current_names = current_names{1};
      |     numios = length(current_names);
      |     if length(current_bins) ~= numios,
      |         error('%d field names specified, but %d binary pts?', numios, length(current_bins));
      |     end
      | end
  updebug : Subsystem
      mask Display: fprintf('UP\nDEBUG')
  xps : xps_library/XSG core config  Tag=xps:xsg  hw_sys=ROACH2:sx475t  clk_src=sys_clk  ROACH_clk_src=adc0_clk  ROACH2_clk_src=sys_clk  MKDIG_clk_src=sys_clk  clk_rate=228  sample_period=1  synthesis_tool=XST
  tag scope: cnt_rst=global, gbe_timestep=global, spead_data0=global, spead_data1=global, spead_data2=global, spead_data3=global, spead_eof0=global, spead_eof1=global, spead_eof2=global, spead_eof3=global, spead_valid0=global, spead_valid1=global, spead_valid2=global, spead_valid3=global, tvg_select0=global, up_cnt_rst=global
  wires:
  gbe0/1(led_up) -> Inverter/1, [up_gbe0]
  gbe0/2(led_rx) -> [rx_gbe0]
  gbe0/3(led_tx) -> [tx_gbe0]
  gbe0/5(tx_overflow) -> [tx_over_gbe0], [of_xaui0]
  gbe0/12(rx_overrun) -> [rxover_gbe0]
  gbe0/11(rx_bad_frame) -> [rxbad_gbe0]
  gbe0/6(rx_data) -> [rxdata_gbe0]
  gbe0/7(rx_valid) -> [rxvld_gbe0]
  gbe0/8(rx_source_ip) -> [rxip_gbe0]
  gbe0/9(rx_source_port) -> [rxport_gbe0]
  gbe0/10(rx_end_of_frame) -> [rxeof_gbe0]
  Inverter/1 -> [ldn_xaui0]
  [gbe_rst] -> Delay12/1
  gbe1/1(led_up) -> [up_gbe1], Inverter1/1
  gbe1/2(led_rx) -> [rx_gbe1]
  gbe1/3(led_tx) -> [tx_gbe1]
  gbe1/4(tx_afull) -> [tx_full_gbe1]
  gbe1/5(tx_overflow) -> [tx_over_gbe1], [of_xaui1]
  gbe1/12(rx_overrun) -> [rxover_gbe1]
  gbe1/11(rx_bad_frame) -> [rxbad_gbe1]
  gbe1/6(rx_data) -> [rxdata_gbe1]
  gbe1/7(rx_valid) -> [rxvld_gbe1]
  gbe1/8(rx_source_ip) -> [rxip_gbe1]
  gbe1/9(rx_source_port) -> [rxport_gbe1]
  gbe1/10(rx_end_of_frame) -> [rxeof_gbe1]
  Inverter1/1 -> [ldn_xaui1]
  Delay12/1 -> gbe1/1(rst)
  gbe2/1(led_up) -> [up_gbe2], Inverter3/1
  gbe2/2(led_rx) -> [rx_gbe2]
  gbe2/3(led_tx) -> [tx_gbe2]
  gbe2/4(tx_afull) -> [tx_full_gbe2]
  gbe2/5(tx_overflow) -> [tx_over_gbe2], [of_xaui2]
  gbe2/12(rx_overrun) -> [rxover_gbe2]
  gbe2/11(rx_bad_frame) -> [rxbad_gbe2]
  gbe2/6(rx_data) -> [rxdata_gbe2]
  gbe2/7(rx_valid) -> [rxvld_gbe2]
  gbe2/8(rx_source_ip) -> [rxip_gbe2]
  gbe2/9(rx_source_port) -> [rxport_gbe2]
  gbe2/10(rx_end_of_frame) -> [rxeof_gbe2]
  Inverter3/1 -> [ldn_xaui2]
  gbe3/1(led_up) -> [up_gbe3], Inverter4/1
  gbe3/2(led_rx) -> [rx_gbe3]
  gbe3/3(led_tx) -> [tx_gbe3]
  gbe3/4(tx_afull) -> [tx_full_gbe3]
  gbe3/5(tx_overflow) -> [tx_over_gbe3], [of_xaui3]
  gbe3/12(rx_overrun) -> [rxover_gbe3]
  gbe3/11(rx_bad_frame) -> [rxbad_gbe3]
  gbe3/6(rx_data) -> [rxdata_gbe3]
  gbe3/7(rx_valid) -> [rxvld_gbe3]
  gbe3/8(rx_source_ip) -> [rxip_gbe3]
  gbe3/9(rx_source_port) -> [rxport_gbe3]
  gbe3/10(rx_end_of_frame) -> [rxeof_gbe3]
  Inverter4/1 -> [ldn_xaui3]
  gbe0/4(tx_afull) -> [tx_full_gbe0]
  bus_expand1/2(lsb_out1) -> aligned/2, misaligned/2
  bus_expand1/1(msb_out2) -> misaligned/1, aligned/1
  aligned/1 -> Register4/1
  misaligned/1 -> Register5/1
  [clr_status] -> Register5/2, Register4/2
  Register5/1 -> [data_misaligned]
  Register4/1 -> [data_aligned]
  edge_detect3/1(out) -> pipeline4/1(d)
  edge_detect4/1(out) -> pipeline3/1(d)
  edge_detect5/1(out) -> pipeline2/1(d)
  [unpack_en] -> Register5/3, Register4/3
  [unpack_recvd] -> bus_expand1/1(bus_in)
  Delay8/1 -> [unpack_d80]
  Delay59/1 -> [unpack_en]  "re80_v"
  Delay62/1 -> aligned1/1
  Delay71/1 -> aligned1/2
  Delay78/1 -> [unpack_recvd]
  [sys_rst] -> edge_detect9/1(in)
  [rxdata_gbe0] -> concat0/1
  [rxdata_gbe1] -> concat0/2
  [rxdata_gbe2] -> concat0/3
  [rxdata_gbe3] -> concat0/4
  [rxeof_gbe0] -> concat1/1
  [rxeof_gbe1] -> concat1/2
  [rxeof_gbe2] -> concat1/3
  [rxeof_gbe3] -> concat1/4
  [rxvld_gbe0] -> concat3/1
  [rxvld_gbe1] -> concat3/2
  [rxvld_gbe2] -> concat3/3
  [rxvld_gbe3] -> concat3/4
  bus_expand2/1(msb_out2) -> Delay62/1
  bus_expand2/2(lsb_out1) -> Delay71/1
  control/2(in_arm) -> edge_detect5/1(in)
  Delay82/1 -> [unpack_timestamp]  "tstamp"
  control/13(in_cnt_rst) -> edge_detect1/1(in)
  concat0/1 -> Delay30/1
  concat1/1 -> Delay31/1
  concat3/1 -> Delay32/1
  constant/1 -> unpack_and_reorder/5(transmit)
  unpack_and_reorder/4(timestamp) -> Delay82/1
  unpack_and_reorder/5(recvd) -> Delay78/1
  unpack_and_reorder/6(of_count) -> bus_expand2/1(bus_in)
  unpack_and_reorder/1(sync) -> Delay41/1
  unpack_and_reorder/7(fifo_of) -> [unpack_fifo_or]
  edge_detect1/1(out) -> pipeline14/1(d)
  control/4(in_gbe_rst) -> pipeline5/1(d)
  control/1(in_sys_rst) -> pipeline/1(d)
  Constant4/1 -> gbe1/8(rx_overrun_ack), gbe1/7(rx_ack)
  [gbe_rst] -> Delay10/1
  Delay10/1 -> gbe2/1(rst)
  Constant23/1 -> gbe2/8(rx_overrun_ack), gbe2/7(rx_ack)
  [gbe_rst] -> Delay11/1
  Delay11/1 -> gbe3/1(rst)
  Constant33/1 -> gbe3/8(rx_overrun_ack), gbe3/7(rx_ack)
  [gbe_rst] -> Delay14/1
  [spead_data0] -> Delay24/1
  [gbe_ip0] -> Delay25/1
  [gbe_port0] -> Delay26/1
  Logical2/1 -> gbe0/3(tx_valid)
  Constant20/1 -> gbe0/8(rx_overrun_ack), gbe0/7(rx_ack)
  [gbe_cnt_rst] -> Delay47/1
  [gbe_cnt_rst] -> Delay46/1
  [gbe_cnt_rst] -> Delay45/1
  [gbe_cnt_rst] -> Delay44/1
  [gbe_txen] -> Logical4/2, Logical2/2
  [spead_valid0] -> Logical2/1
  [spead_data1] -> Delay27/1
  [gbe_ip1] -> Delay28/1
  [gbe_port1] -> Delay33/1
  [gbe_txen] -> Logical3/2, Logical7/2
  [spead_valid1] -> Logical7/1
  Logical7/1 -> gbe1/3(tx_valid)
  [spead_data2] -> Delay35/1
  [gbe_ip2] -> Delay36/1
  [gbe_port2] -> Delay37/1
  [gbe_txen] -> Logical11/2, Logical8/2
  [spead_valid2] -> Logical8/1
  [spead_data3] -> Delay38/1
  [gbe_ip3] -> Delay39/1
  [gbe_port3] -> Delay40/1
  [gbe_txen] -> Logical12/2, Logical9/2
  [spead_valid3] -> Logical9/1
  Logical8/1 -> gbe2/3(tx_valid)
  Logical9/1 -> gbe3/3(tx_valid)
  pipeline/1(q) -> [sys_rst]
  pipeline2/1(q) -> [arm]
  pipeline3/1(q) -> [clr_status]
  pipeline4/1(q) -> [clr_adc_bad]
  pipeline5/1(q) -> [gbe_rst]
  pipeline6/1(q) -> [gbe_txen]
  pipeline8/1(q) -> [adc_protect_disable]
  pipeline9/1(q) -> [tvg_en]
  pipeline10/1(q) -> [ct_tvg]
  pipeline11/1(q) -> [packetiser_tvg]
  pipeline12/1(q) -> [fd_fs_tvg]
  pipeline13/1(q) -> [tvg_adc_en]
  pipeline14/1(q) -> [cnt_rst]
  control/12(in_tvg_adc) -> pipeline13/1(d)
  unpack_and_reorder/8(packet_of) -> [fifo_pktof]
  Delay29/1 -> unpack_and_reorder/1(rst)
  Delay30/1 -> unpack_and_reorder/2(din)
  Delay31/1 -> unpack_and_reorder/3(eof)
  Delay32/1 -> unpack_and_reorder/4(en)
  Delay44/1 -> gbe3/9(debug_rst)
  Delay45/1 -> gbe2/9(debug_rst)
  Delay46/1 -> gbe1/9(debug_rst)
  Delay47/1 -> gbe0/9(debug_rst)
  edge_detect2/1(out) -> pipeline7/1(d)
  pipeline7/1(q) -> [gbe_cnt_rst]
  control/14(in_gbe_cnt_rst) -> edge_detect2/1(in)
  Logical3/1 -> gbe1/6(tx_end_of_frame)
  [spead_eof1] -> Logical3/1
  Logical4/1 -> gbe0/6(tx_end_of_frame)
  [spead_eof0] -> Logical4/1
  Logical11/1 -> gbe2/6(tx_end_of_frame)
  [spead_eof2] -> Logical11/1
  Logical12/1 -> gbe3/6(tx_end_of_frame)
  [spead_eof3] -> Logical12/1
  Delay14/1 -> gbe0/1(rst)
  edge_detect7/1(out) -> pipeline15/1(d)
  pipeline15/1(q) -> [up_cnt_rst]
  Delay24/1 -> gbe0/2(tx_data)
  Delay25/1 -> gbe0/4(tx_dest_ip)
  Delay26/1 -> gbe0/5(tx_dest_port)
  Delay27/1 -> gbe1/2(tx_data)
  Delay28/1 -> gbe1/4(tx_dest_ip)
  Delay33/1 -> gbe1/5(tx_dest_port)
  Delay35/1 -> gbe2/2(tx_data)
  Delay36/1 -> gbe2/4(tx_dest_ip)
  Delay37/1 -> gbe2/5(tx_dest_port)
  Delay38/1 -> gbe3/2(tx_data)
  Delay39/1 -> gbe3/4(tx_dest_ip)
  Delay40/1 -> gbe3/5(tx_dest_port)
  unpack_and_reorder/2(dout) -> Delay8/1
  unpack_and_reorder/3(dvalid) -> Delay59/1
  unpack_and_reorder/9(spead_error) -> Terminator1/1
  unpack_and_reorder/10(discarding) -> Terminator2/1
  unpack_and_reorder/11(timestep_error) -> [timestep_error]
  [unpack_en] -> en_gen/2(en)
  [unpack_timestamp] -> en_gen/3(time_in)
  en_gen/1(dout) -> sync_gen/1(din)
  sync_gen/1(sync) -> data_tvg1/2(sync_in), data_tvg0/2(sync_in)
  data_tvg0/3(dvalid) -> [valid80]
  data_tvg0/1(sync_out) -> [sync80]
  bus_expand6/2(lsb_out1) -> data_tvg1/3(din)
  data_tvg0/2(dout) -> [d80_adc0]
  [tvg_d80_en] -> en_gen/5(tvg_en)
  [unpack_d80] -> en_gen/1(din)
  bus_expand6/1(msb_out2) -> data_tvg0/3(din)
  data_tvg0/4(misco) -> [time80]
  sync_gen/5(misco) -> data_tvg1/5(misci)
  data_tvg1/2(dout) -> [d80_adc1]
  data_tvg1/3(dvalid) -> [valid80_1]
  data_tvg1/1(sync_out) -> Terminator4/1
  Concat/1 -> en_gen/4(misci)
  [unpack_adc_or] -> Concat/1
  [data_misaligned] -> Concat/2
  data_tvg1/4(misco) -> bus_expand19/1(bus_in)
  bus_expand19/1(msb_out2) -> [adc_or_flag]
  bus_expand19/2(lsb_out1) -> [missing_flag]
  [tvg_adc_en] -> data_tvg0/1(tvg_en), data_tvg1/1(tvg_en)
  en_gen/3(time_out) -> sync_gen/3(time_in)
  en_gen/2(dvalid) -> sync_gen/2(en)
  en_gen/4(misco) -> Slice20/1, Slice19/1
  Slice19/1 -> sync_gen/4(misci)
  Slice20/1 -> sync_gen/5(relock)
  sync_gen/4(time_out) -> data_tvg0/5(misci)
  sync_gen/2(dout) -> bus_expand6/1(bus_in)
  sync_gen/3(dvalid) -> data_tvg1/4(en), data_tvg0/4(en)
  [timestep_error] -> Concat/3
  Slice/1 -> pipeline16/1(d)
  pipeline16/1(q) -> local_time_lsw/1(out_timestamp_lsw)
  Slice16/1 -> Convert1/1
  pipeline47/1(q) -> local_time_msw/1(out_timestamp_msw)
  Convert1/1 -> pipeline47/1(d)
  Concat2/1 -> Slice16/1, [time80_48], Slice/1
  [time80] -> Concat2/1
  Constant53/1 -> Concat2/2
  control/15(in_unpack_cnt_rst) -> edge_detect7/1(in)
  pipeline18/1(q) -> [snappfb_arm]
  control/17(in_snappfb_arm) -> pipeline18/1(d)
  control/5(in_gbe_txen) -> pipeline6/1(d)
  control/6(in_adc_bad_clr) -> edge_detect3/1(in)
  control/7(in_adc_protect_disable) -> pipeline8/1(d)
  control/8(in_tvg_en) -> pipeline9/1(d)
  control/9(in_tvg_ct) -> pipeline10/1(d)
  control/10(in_tvg_packetiser) -> pipeline11/1(d)
  control/11(in_tvg_fdfs) -> pipeline12/1(d)
  pipeline19/1(q) -> [tvg_d80_en]
  control/20(in_tvg_d80) -> pipeline19/1(d)
  aligned1/1 -> [unpack_adc_or]
  control/3(in_status_clr) -> edge_detect4/1(in)
  Delay41/1 -> [unpack_sync]
  Register11/1 -> Slice9/1, Slice7/1
  [time80] -> pipeline54/1(d)
  Slice7/1 -> sync_timestamp_msw/1(out_reg)
  [sync80] -> pipeline52/1(d)
  [valid80] -> pipeline53/1(d)
  Register12/1 -> Logical1/1  "armed"
  Logical1/1 -> Register12/2, Register11/2
  pipeline52/1(q) -> Register12/3, Register12/1
  pipeline53/1(q) -> Logical1/2
  pipeline54/1(q) -> Register11/1
  [valid80] -> pipeline55/1(d)
  pipeline55/1(q) -> Delay42/1, edge_detect13/1(in)
  counter8/1 -> Register13/1
  edge_detect13/1(out) -> counter8/1, Register13/2
  Delay42/1 -> counter8/2
  Slice9/1 -> sync_timestamp_lsw/1(out_time_lsw)
  Register13/1 -> sync_timestamp_lsw/2(out_pkt_size)
  pipeline56/1(q) -> edge_detect14/1(in)
  edge_detect14/1(out) -> counter9/2
  [timestep_error] -> pipeline56/1(d)
  [cnt_rst] -> pipeline57/1(d)
  pipeline57/1(q) -> counter9/1
  pipeline58/1(q) -> edge_detect15/1(in)
  edge_detect15/1(out) -> counter10/2
  [sync80] -> pipeline58/1(d)
  [cnt_rst] -> pipeline51/1(d)
  pipeline51/1(q) -> counter10/1
  pipeline59/1(q) -> edge_detect16/1(in)
  edge_detect16/1(out) -> counter11/2
  [valid80] -> pipeline59/1(d)
  [cnt_rst] -> pipeline60/1(d)
  pipeline60/1(q) -> counter11/1
  counter9/1 -> sync_timestamp_lsw/3(out_tstep_err_ctr)
  counter10/1 -> sync_timestamp_lsw/4(out_sync80_ctr)
  counter11/1 -> sync_timestamp_lsw/5(out_valid80_ctr)
  pipeline48/1(q) -> [tvg_select0]
  edge_detect9/1(out) -> Delay29/1
  [up_p0_missed_time_ctr] -> Delay76/1(d)
  [up_p1_missed_time_ctr] -> Delay77/1(d)
  [up_p0_missed_time] -> Delay81/1(d)
  [up_p1_missed_time] -> Delay83/1(d)
  Delay81/1(q) -> Slice10/1
  Delay83/1(q) -> Slice11/1
  Delay76/1(q) -> tmiss_ctr/1(out_p0)
  Delay77/1(q) -> tmiss_ctr/2(out_p1)
  [unpack_recvd] -> Slice17/1, Slice12/1
  Inverter2/1 -> Logical5/1
  [unpack_en] -> Logical6/2, Logical5/2
  Logical5/1 -> counter20/2
  [cnt_rst] -> Delay79/1(d)
  counter20/1 -> recverr_ctr/1(out_p0)
  counter21/1 -> mcnt_relock/1(out_reg)
  [mcnt_relock] -> counter21/2
  Slice10/1 -> tmiss_p0/1(out_reg)
  Slice11/1 -> tmiss_p1/1(out_reg)
  counter22/1 -> recverr_ctr/2(out_p1)
  Slice12/1 -> Inverter2/1
  Logical6/1 -> counter22/2
  Slice17/1 -> Inverter5/1
  Inverter5/1 -> Logical6/1
  [up_timestep_error_future] -> counter23/2
  [up_timestep_error_past] -> counter13/2
  Delay79/1(q) -> counter22/1, counter23/1, counter13/1, counter21/1, counter20/1
  counter23/1 -> timestep_ages/1(out_future)
  counter13/1 -> timestep_ages/2(out_past)
  pipeline67/1(q) -> [snappfb_dsel]
  control/18(in_snappfb_dsel) -> pipeline67/1(d)
  pipeline72/1(q) -> [snapcoarse_arm]
  control/16(in_snapcoarse_arm) -> pipeline72/1(d)
  pipeline77/1(q) -> [snapquant_arm]
  control/19(in_snapquant_arm) -> pipeline77/1(d)
  [up_gbe0] -> gbe_status/1(out_gbe0_linkup)
  [up_gbe1] -> gbe_status/2(out_gbe1_linkup)
  [up_gbe2] -> gbe_status/3(out_gbe2_linkup)
  [up_gbe3] -> gbe_status/4(out_gbe3_linkup)
  up_debug/1(in_gbe_timestep) -> Delay88/1(d)
  Delay88/1(q) -> [gbe_timestep]
  unpack_and_reorder/12(mcnt_relock) -> [mcnt_relock]
  [sync80] -> pipeline1/1(d)
  [valid80] -> pipeline17/1(d)
  bus_expand3/1(msb_out8) -> dec_fir_async/3(real1)
  bus_expand3/2(out7) -> dec_fir_async/5(real2)
  bus_expand3/3(out6) -> dec_fir_async/7(real3)
  bus_expand3/4(out5) -> dec_fir_async/9(real4)
  bus_expand3/5(out4) -> dec_fir_async/11(real5)
  bus_expand3/6(out3) -> dec_fir_async/13(real6)
  bus_expand3/7(out2) -> dec_fir_async/15(real7)
  bus_expand3/8(lsb_out1) -> dec_fir_async/17(real8)
  bus_expand4/8(lsb_out1) -> dec_fir_async/18(imag8)
  bus_expand4/7(out2) -> dec_fir_async/16(imag7)
  bus_expand4/6(out3) -> dec_fir_async/14(imag6)
  bus_expand4/5(out4) -> dec_fir_async/12(imag5)
  bus_expand4/4(out5) -> dec_fir_async/10(imag4)
  bus_expand4/3(out6) -> dec_fir_async/8(imag3)
  bus_expand4/2(out7) -> dec_fir_async/6(imag2)
  bus_expand4/1(msb_out8) -> dec_fir_async/4(imag1)
  [d80_adc0] -> pipeline20/1(d)
  [d80_adc1] -> pipeline21/1(d)
  [sync_filt] -> serial_to_8par1/1(sync), serial_to_8par/1(sync)
  serial_to_8par/1(sync_out) -> [sync_f80]
  serial_to_8par/2(dv_out) -> [dv_f80]
  serial_to_8par/3(data0_old) -> Concat1/1
  serial_to_8par/4(data1) -> Concat1/2
  serial_to_8par/5(data2) -> Concat1/3
  serial_to_8par/6(data3) -> Concat1/4
  serial_to_8par/7(data4) -> Concat1/5
  serial_to_8par/8(data5) -> Concat1/6
  serial_to_8par/9(data6) -> Concat1/7
  serial_to_8par/10(data7_new) -> Concat1/8
  dec_fir_async/1(sync_out) -> [sync_filt]
  dec_fir_async/2(dout) -> bus_expand5/1(bus_in)
  bus_expand5/1(msb_out2) -> [d10_filt_0]
  bus_expand5/2(lsb_out1) -> [d10_filt_1]
  dec_fir_async/3(dv_out) -> [dv_filt]
  pipeline1/1(q) -> dec_fir_async/1(sync_in)
  pipeline17/1(q) -> dec_fir_async/2(dv_in)
  pipeline20/1(q) -> bus_expand3/1(bus_in)
  pipeline21/1(q) -> bus_expand4/1(bus_in)
  [d10_filt_0] -> serial_to_8par/3(data)
  [dv_filt] -> serial_to_8par1/2(dv), serial_to_8par/2(dv)
  [d10_filt_1] -> serial_to_8par1/3(data)
  serial_to_8par1/1(sync_out) -> Terminator/1
  serial_to_8par1/2(dv_out) -> Register3/2, Terminator3/1
  serial_to_8par1/9(data6) -> Concat3/7
  serial_to_8par1/8(data5) -> Concat3/6
  serial_to_8par1/10(data7_new) -> Concat3/8
  serial_to_8par1/3(data0_old) -> Concat3/1
  serial_to_8par1/4(data1) -> Concat3/2
  serial_to_8par1/5(data2) -> Concat3/3
  serial_to_8par1/6(data3) -> Concat3/4
  serial_to_8par1/7(data4) -> Concat3/5
  Concat1/1 -> [d_f80_0]
  Concat3/1 -> [d_f80_1]
  [cnt_rst] -> pipeline22/1(d)
  pipeline22/1(q) -> counter1/1
  Logical10/1 -> counter1/2
  [valid80] -> Logical10/1
  [valid80_1] -> Logical10/2
  counter1/1 -> dv_misaligned/1(out_reg)
  [d_f80_0] -> Mux/3, Mux/4, Mux/2
  [tvg_select0] -> Mux/1
  Mux/1 -> Assert/1  "d80_0"
  fifo0/1(fifo_data80) -> pack_80_64_00/1(data80)  "data00"
  fifo0/2(fifo_dv) -> pack_80_64_00/2(valid80)  "dv00"
  fifo0/3(word_start) -> pack_80_64_00/3(word_start)  "ws00"
  fifo0/4(pkt_start) -> pack_80_64_00/4(pkt_start)  "ps00"
  fifo0/5(fifo_full) -> Terminator16/1  "full00"
  fifo0/6(fifo_empty) -> Terminator23/1  "empty00"
  fifo1/1(fifo_data80) -> pack_80_64_01/1(data80)  "data01"
  fifo1/2(fifo_dv) -> pack_80_64_01/2(valid80)  "dv01"
  fifo1/3(word_start) -> pack_80_64_01/3(word_start)  "ws01"
  fifo1/4(pkt_start) -> pack_80_64_01/4(pkt_start)  "ps01"
  pack_80_64_01/3(data64) -> spead_pack1/3(data64)  "d64_00"
  pack_80_64_01/2(valid64) -> spead_pack1/2(data64_valid)  "v64_01"
  pack_80_64_01/1(ready64) -> spead_pack1/1(data64_ready)  "r64_01"
  fifo1/5(fifo_full) -> Terminator18/1
  fifo1/6(fifo_empty) -> Terminator20/1
  Inverter6/1 -> fifo1/2(fifo_we_en)
  [hdr_0x3101] -> bus_create9/1(in1)
  [pol0_id] -> bus_create9/2(in2)
  [hdr_0x3101] -> bus_create1/1(in1)
  [pol0_id] -> bus_create1/2(in2)
  [speadtime0] -> spead_pack0/8(hdr5_0x1600_DIR), spead_pack0/4(hdr_heap_id)  "timein0"
  bus_create9/1(bus_out) -> spead_pack0/9(hdr6_0x3101_DIR)
  [status0] -> spead_pack0/10(hdr7_0x3102_DIR)
  bus_create1/1(bus_out) -> spead_pack1/9(hdr6_0x3101_DIR)
  [status1] -> spead_pack1/10(hdr7_0x3102_DIR)
  fifo_select/1(select) -> Delay3/1  "fifo_select"
  Delay3/1 -> [fifoselect], Inverter6/1, fifo0/2(fifo_we_en)  "fifoselect"
  [speadtime1] -> spead_pack1/4(hdr_heap_id), spead_pack1/8(hdr5_0x1600_DIR)  "timein1"
  pack_80_64_00/1(ready64) -> spead_pack0/1(data64_ready)  "r64_00"
  pack_80_64_00/2(valid64) -> spead_pack0/2(data64_valid)  "v64_00"
  pack_80_64_00/3(data64) -> spead_pack0/3(data64)  "d64_00"
  [spead_heapsize] -> spead_pack0/5(hdr_heap_size)
  [spead_heapoffset] -> spead_pack0/6(hdr_heap_offset)
  [spead_pktlen] -> spead_pack0/7(hdr_pkt_len_words)
  [spead_heapsize] -> spead_pack1/5(hdr_heap_size)
  [spead_heapoffset] -> spead_pack1/6(hdr_heap_offset)
  [spead_pktlen] -> spead_pack1/7(hdr_pkt_len_words)
  Assert/1 -> bus_expand7/1(bus_in), fifo1/1(data80), fifo0/1(data80)
  spead_pack1/4(data_overflow) -> Terminator15/1
  [adc_data_offset] -> spead_pack0/11(hdr8_0x3300)
  [adc_data_offset] -> spead_pack1/11(hdr8_0x3300)
  Constant26/1 -> [spead_heapsize]
  Constant27/1 -> [spead_pktlen]
  Constant45/1 -> [spead_heapoffset]
  bus_expand7/1(msb_out3) -> Terminator50/1  "pkt_time"
  bus_expand7/2(out2) -> Terminator51/1  "pkt_ctr"
  bus_expand7/3(lsb_out1) -> Terminator49/1  "pkt_pol"
  spead_pack0/4(data_overflow) -> Terminator12/1
  spead_pack0/3(eof) -> [spead_eof0]
  spead_pack0/1(data_out) -> [spead_data0]  "packd"
  spead_pack0/2(valid_out) -> [spead_valid0]  "packv"
  spead_pack1/1(data_out) -> [spead_data1]
  spead_pack1/2(valid_out) -> [spead_valid1]
  spead_pack1/3(eof) -> [spead_eof1]
  Delay4/1 -> Register6/1, Register1/1  "tvgtime"
  [fifoselect] -> Inverter8/1, edge_detect6/1(in)
  Register1/1 -> [speadtime0]  "speadtime0"
  Inverter8/1 -> edge_detect8/1(in)
  edge_detect6/1(out) -> Register1/2
  edge_detect8/1(out) -> Register6/2
  Register6/1 -> [speadtime1]  "speadtime1"
  slice1/1 -> fifo_select/1(localtime)
  Constant8/1 -> [adc_data_offset]
  fifo2/1(fifo_data80) -> pack_80_64_1/1(data80)  "data00"
  fifo2/2(fifo_dv) -> pack_80_64_1/2(valid80)  "dv00"
  fifo2/3(word_start) -> pack_80_64_1/3(word_start)  "ws00"
  fifo2/4(pkt_start) -> pack_80_64_1/4(pkt_start)  "ps00"
  fifo2/5(fifo_full) -> Terminator7/1  "full00"
  fifo2/6(fifo_empty) -> Terminator10/1  "empty00"
  fifo3/1(fifo_data80) -> pack_80_64_2/1(data80)  "data01"
  fifo3/2(fifo_dv) -> pack_80_64_2/2(valid80)  "dv01"
  fifo3/3(word_start) -> pack_80_64_2/3(word_start)  "ws01"
  fifo3/4(pkt_start) -> pack_80_64_2/4(pkt_start)  "ps01"
  pack_80_64_2/3(data64) -> spead_pack3/3(data64)  "d64_00"
  pack_80_64_2/2(valid64) -> spead_pack3/2(data64_valid)  "v64_01"
  pack_80_64_2/1(ready64) -> spead_pack3/1(data64_ready)  "r64_01"
  fifo3/5(fifo_full) -> Terminator8/1
  fifo3/6(fifo_empty) -> Terminator9/1
  [hdr_0x3101] -> bus_create3/1(in1)
  [pol1_id] -> bus_create3/2(in2)
  [hdr_0x3101] -> bus_create2/1(in1)
  [pol1_id] -> bus_create2/2(in2)
  [speadtime0] -> spead_pack2/4(hdr_heap_id), spead_pack2/8(hdr5_0x1600_DIR)  "timein0"
  bus_create3/1(bus_out) -> spead_pack2/9(hdr6_0x3101_DIR)
  [status2] -> spead_pack2/10(hdr7_0x3102_DIR)
  bus_create2/1(bus_out) -> spead_pack3/9(hdr6_0x3101_DIR)
  [status3] -> spead_pack3/10(hdr7_0x3102_DIR)
  [speadtime1] -> spead_pack3/8(hdr5_0x1600_DIR), spead_pack3/4(hdr_heap_id)  "timein1"
  pack_80_64_1/1(ready64) -> spead_pack2/1(data64_ready)  "r64_00"
  pack_80_64_1/2(valid64) -> spead_pack2/2(data64_valid)  "v64_00"
  pack_80_64_1/3(data64) -> spead_pack2/3(data64)  "d64_00"
  [spead_heapsize] -> spead_pack2/5(hdr_heap_size)
  [spead_heapoffset] -> spead_pack2/6(hdr_heap_offset)
  [spead_pktlen] -> spead_pack2/7(hdr_pkt_len_words)
  [spead_heapsize] -> spead_pack3/5(hdr_heap_size)
  [spead_heapoffset] -> spead_pack3/6(hdr_heap_offset)
  [spead_pktlen] -> spead_pack3/7(hdr_pkt_len_words)
  spead_pack3/4(data_overflow) -> Terminator6/1
  [adc_data_offset] -> spead_pack2/11(hdr8_0x3300)
  [adc_data_offset] -> spead_pack3/11(hdr8_0x3300)
  spead_pack2/4(data_overflow) -> Terminator5/1
  spead_pack2/3(eof) -> [spead_eof2]
  spead_pack2/1(data_out) -> [spead_data2]  "packd"
  spead_pack2/2(valid_out) -> [spead_valid2]  "packv"
  spead_pack3/1(data_out) -> [spead_data3]
  spead_pack3/2(valid_out) -> [spead_valid3]
  spead_pack3/3(eof) -> [spead_eof3]
  Inverter7/1 -> fifo3/2(fifo_we_en)
  [d_f80_1] -> Mux1/3, Mux1/4, Mux1/2
  [tvg_select0] -> Mux1/1
  Mux1/1 -> Assert1/1  "d80_0"
  Assert1/1 -> fifo3/1(data80), fifo2/1(data80)
  [fifoselect] -> Inverter7/1, fifo2/2(fifo_we_en)
  tvgsel/1(in_tvgsel) -> pipeline48/1(d)
  [time80_48] -> pipeline23/1(d)
  pipeline23/1(q) -> [time48_filt]
  Register3/1 -> [time48_f80]
  [time48_filt] -> Register3/1
  [time48_f80] -> Delay4/1, slice1/1
  gbe_porttx/1(in_reg) -> [gbe_port0], [gbe_port1], [gbe_port2], [gbe_port3]
  gbe_iptx0/1(in_reg) -> [gbe_ip0]
  gbe_iptx1/1(in_reg) -> [gbe_ip1]
  gbe_iptx2/1(in_reg) -> [gbe_ip2]
  gbe_iptx3/1(in_reg) -> [gbe_ip3]
  Constant9/1 -> gbe_porttx/1(sim_1)
  Constant10/1 -> gbe_iptx0/1(sim_1)
  Constant12/1 -> gbe_iptx1/1(sim_1)
  Constant13/1 -> gbe_iptx2/1(sim_1)
  Constant14/1 -> gbe_iptx3/1(sim_1)
  Constant15/1 -> digitiser_id/1(sim_1)
  Constant17/1 -> receptor_id/1(sim_1)
  bus_create/1(bus_out) -> [hdr_0x3101]
  Constant16/1 -> digitiser_id/2(sim_2)
  receptor_id/1(in_receptor_id) -> bus_create/3(in3)
  receptor_id/2(in_pol0_id) -> [pol0_id]
  receptor_id/3(in_pol1_id) -> [pol1_id]
  Constant6/1 -> receptor_id/2(sim_2)
  Constant19/1 -> receptor_id/3(sim_3)
  digitiser_id/1(in_digitiser_serial) -> bus_create/1(in1)
  digitiser_id/2(in_digitiser_type) -> bus_create/2(in2)
  Constant1/1 -> [status3], [status2], [status1], [status0]  "status"
